simulink library "dlbsBlockInsertGradientGF"  (R2025b)
settings: Solver=VariableStepAuto  StartTime=0.0  StopTime=10.0  RelTol=1e-3
settings Model: Creator=lt6037  LastModifiedBy=lt6037

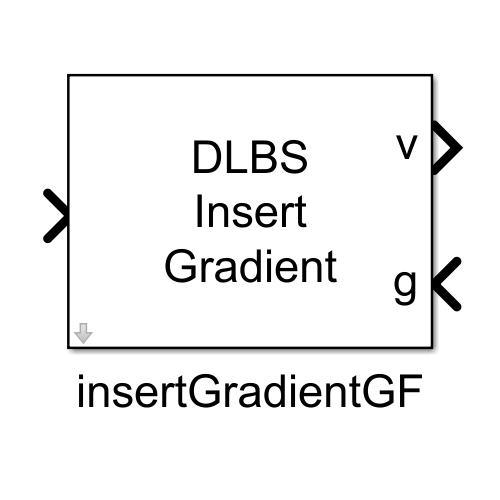
[thumbnail: Simulink's stored preview of the top-level diagram]
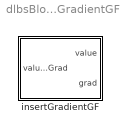
== system dlbsBlockInsertGradientGF ==
  insertGradientGF : Subsystem
      settings: PortSchema="{\"entries\":[{\"content\":{\"sides\":[{\"content\":{\"connectorIds\":[\"In1\"]},\"type\":\"ConnectorPlacement.EquallySpacedRectSide\",\"uuid\":\"7478b886-f2f3-470d-a9fc-eb7d3f1c7d28\"},{\"content\":{\"connectorIds\":[\"Out1\",\"In2\"],\"side\":\"RIGHT\"},\"type\":\"ConnectorPlacement.EquallySpacedRectSide\",\"uuid\":\"d9c780f7-90e1-4769-bdc4-acf73b32d815\"},{\"content\":{\"side\":\"TOP\"},\"type\":\"ConnectorPlacement.EquallySpacedRectSide\",\"uuid\":\"49524ff5-2569-4f81-9b54-143f15fd4d00\"}]},\"type\":\"ConnectorPlacement.EquallySpacedConnector\",\"uuid\":\"bfc235a9-1f2d-4e7e-a59f-bc5a03e5ab10\"}],\"packageUris\":[\"http://schema.mathworks.com/mf0/Connector/R2020b\"],\"version\":\"1.0\"}"
      mask Display:
      | % val
      | port_label('output', 1, 'v');
      | %val + grad
      | port_label('input', 1, '');
      | % grad
      | port_label('input', 2, 'g');
      | disp("DLBS\nInsert\nGradient")

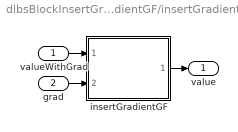
== system dlbsBlockInsertGradientGF/insertGradientGF ==
  valueWithGrad : Inport
  grad : Inport  Port=2
  insertGradientGF : Subsystem  ReferencedSubsystem=dlbsSubsystemInsertGradientGF
  value : Outport
  wires:
  valueWithGrad/1 -> insertGradientGF/1
  insertGradientGF/1 -> value/1
  grad/1 -> insertGradientGF/2
